simulink model "Simulation_p_controller"  (R2023a)
settings: Solver=VariableStepAuto  StartTime=0.0  StopTime=10.0  MaxStep=1e-3
settings Model: Creator=mazen  LastModifiedBy=mazen

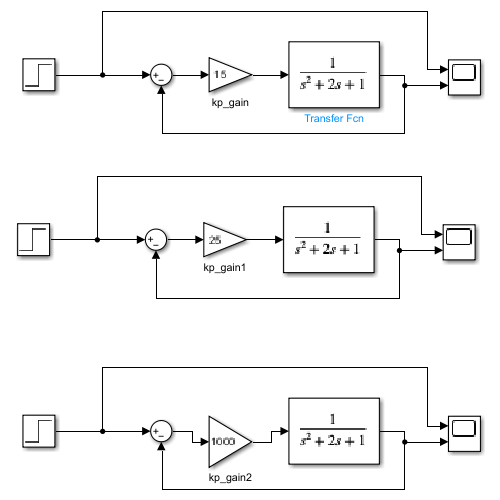
[thumbnail: Simulink's stored preview of the top-level diagram]
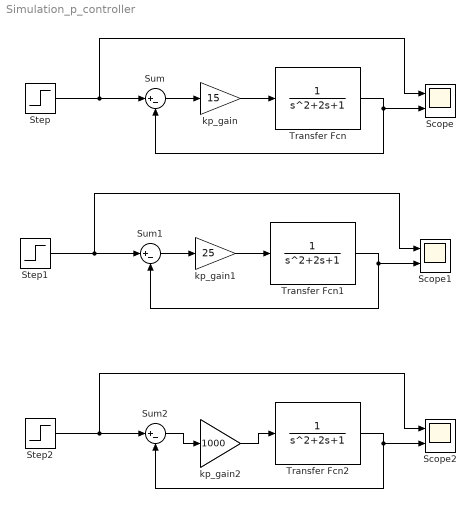
== system Simulation_p_controller ==
  Scope : Scope  NumInputPorts=2
  Scope1 : Scope  NumInputPorts=2
  Scope2 : Scope  NumInputPorts=2
  Step : Step  SampleTime=0
  Step1 : Step  SampleTime=0
  Step2 : Step  SampleTime=0
  Sum : Sum  Inputs=|+-
  Sum1 : Sum  Inputs=|+-
  Sum2 : Sum  Inputs=|+-
  Transfer Fcn : TransferFcn
  Transfer Fcn1 : TransferFcn
  Transfer Fcn2 : TransferFcn
  kp_gain : Gain  Gain=15
  kp_gain1 : Gain  Gain=25
  kp_gain2 : Gain  Gain=1000
  wires:
  Step/1 -> Scope/1, Sum/1
  Transfer Fcn/1 -> Sum/2, Scope/2
  Sum/1 -> kp_gain/1
  kp_gain/1 -> Transfer Fcn/1
  kp_gain1/1 -> Transfer Fcn1/1
  Sum1/1 -> kp_gain1/1
  Transfer Fcn1/1 -> Scope1/2, Sum1/2
  Step1/1 -> Sum1/1, Scope1/1
  Step2/1 -> Scope2/1, Sum2/1
  Transfer Fcn2/1 -> Sum2/2, Scope2/2
  Sum2/1 -> kp_gain2/1
  kp_gain2/1 -> Transfer Fcn2/1
